simulink model "SwitchDemo"  (R2014a)
settings: Solver=ode45  StartTime=0.0  StopTime=10.0  RelTol=1e-3
settings Model: Creator=李广文  LastModifiedBy=李广文

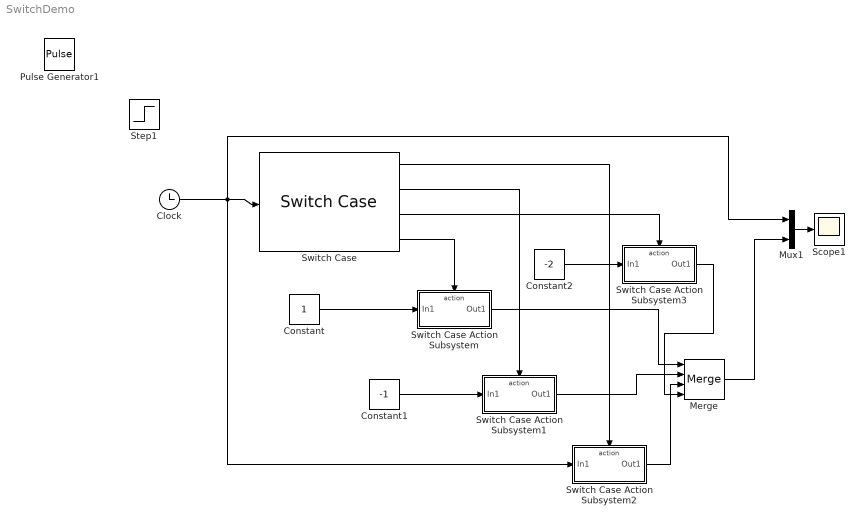
== system SwitchDemo ==
  Clock : Clock
  Constant : Constant
  Constant1 : Constant  Value=-1
  Constant2 : Constant  Value=-2
  Merge : Merge  Inputs=4
  Mux1 : Mux  Inputs=2
  Pulse Generator1 : DiscretePulseGenerator  PulseType=Time based  Period=3  PulseWidth=50
  Scope1 : Scope
      settings: YMin=-2  YMax=2
  Step1 : Step  SampleTime=0
  Switch Case : SwitchCase  CaseConditions={1,[2,3],4}
  Switch Case Action Subsystem : Subsystem  TreatAsAtomicUnit=on
  Switch Case Action Subsystem1 : Subsystem  TreatAsAtomicUnit=on
  Switch Case Action Subsystem2 : Subsystem  TreatAsAtomicUnit=on
  Switch Case Action Subsystem3 : Subsystem  TreatAsAtomicUnit=on
  wires:
  Mux1/1 -> Scope1/1
  Switch Case/4 -> Switch Case Action Subsystem/Action
  Switch Case/2 -> Switch Case Action Subsystem1/Action
  Switch Case/1 -> Switch Case Action Subsystem2/Action
  Constant/1 -> Switch Case Action Subsystem/1(In1)
  Constant1/1 -> Switch Case Action Subsystem1/1(In1)
  Clock/1 -> Mux1/1, Switch Case Action Subsystem2/1(In1), Switch Case/1
  Switch Case Action Subsystem/1(Out1) -> Merge/1
  Switch Case Action Subsystem1/1(Out1) -> Merge/2
  Switch Case Action Subsystem2/1(Out1) -> Merge/3
  Merge/1 -> Mux1/2
  Switch Case/3 -> Switch Case Action Subsystem3/Action
  Constant2/1 -> Switch Case Action Subsystem3/1(In1)
  Switch Case Action Subsystem3/1(Out1) -> Merge/4

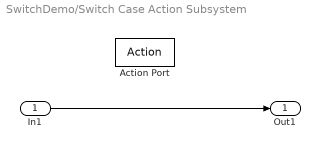
== system SwitchDemo/Switch Case Action Subsystem ==
  In1 : Inport
  Action Port : ActionPort  ActionType=default
  Out1 : Outport
  wires:
  In1/1 -> Out1/1

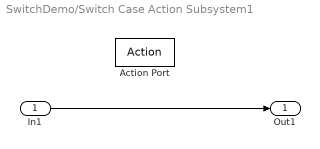
== system SwitchDemo/Switch Case Action Subsystem1 ==
  In1 : Inport
  Action Port : ActionPort  ActionType=case
  Out1 : Outport
  wires:
  In1/1 -> Out1/1

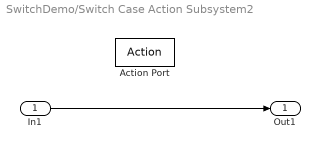
== system SwitchDemo/Switch Case Action Subsystem2 ==
  In1 : Inport
  Action Port : ActionPort  ActionType=case
  Out1 : Outport
  wires:
  In1/1 -> Out1/1

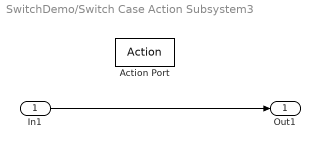
== system SwitchDemo/Switch Case Action Subsystem3 ==
  In1 : Inport
  Action Port : ActionPort  ActionType=case
  Out1 : Outport
  wires:
  In1/1 -> Out1/1
